simulink model "model"  (R2018a)
settings: Solver=FixedStepAuto  StartTime=0.0  StopTime=inf  FixedStep=0.1  MaxStep=0.1  MinStep=0.001  RelTol=1e-3
libraries: vrlib x19, simulink x15
(part 1 of 2)
settings Model: Creator=besho  LastModifiedBy=besho
settings SolverCC: ZeroCrossAlgorithm=Adaptive
settings DataIOCC: SaveOutput=off  SignalLogging=off  DSMLogging=off  SaveTime=off

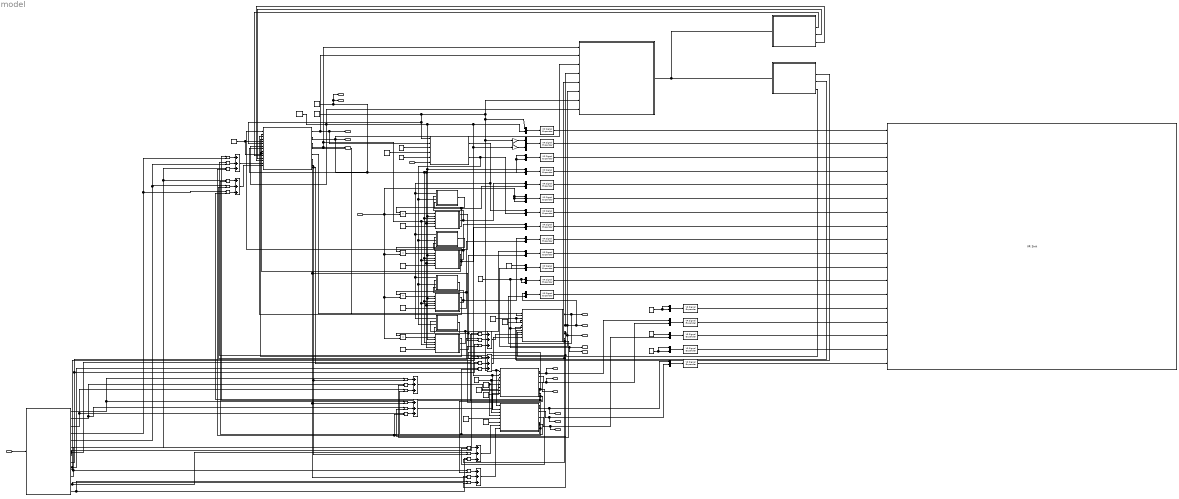
== system model ==
  light_switch : Inport
  light_moving : Inport  Port=2
  collision_matrix : Inport  Port=3  PortDimensions=[4 4]
  Add{,1..7} (8 alike) : Sum  Inputs=+++
  Bus Creator{,1..10,12..17} (17 alike) : BusCreator  Inputs=2
  Bus Creator11 : BusCreator  Inputs=3
  Constant{,1,6,11} (4 alike) : Constant  Value=0
  Constant10 : Constant  Value=200
  Constant{2,12,15..16} (4 alike) : Constant
  Constant13 : Constant  Value=4.7
  Constant14 : Constant  Value=100
  Constant3 : Constant  Value=3*pi/2
  Constant4 : Constant  Value=pi
  Constant5 : Constant  Value=pi/2
  Constant7 : Constant  Value=100
  Constant9 : Constant  Value=3
  Gain : Gain  Gain=1.1
  Gain1 : Gain  Gain=1.1
  MATLAB Function : MATLAB Function  TreatAsAtomicUnit=on
  Multiply{,1..27} (28 alike) : Product
  VR Signal Expander{,1..3,5..8,10,12..13,15..16} (13 alike) : vrlib/VR Signal Expander  outwidth=3  outidx=[1 2]
      settings: SourceProductName=Simulink 3D Animation  SourceProductBaseCode=VR
  VR Signal Expander11 : vrlib/VR Signal Expander  outwidth=3  outidx=[1 2 3]
      settings: SourceProductName=Simulink 3D Animation  SourceProductBaseCode=VR
  VR Signal Expander14 : vrlib/VR Signal Expander  outwidth=3  outidx=[1 3]
      settings: SourceProductName=Simulink 3D Animation  SourceProductBaseCode=VR
  VR Signal Expander17 : vrlib/VR Signal Expander  outwidth=4  outidx=[3 4]
      settings: SourceProductName=Simulink 3D Animation  SourceProductBaseCode=VR
  VR Signal Expander4 : vrlib/VR Signal Expander  outwidth=3  outidx=[1 3]
      settings: SourceProductName=Simulink 3D Animation  SourceProductBaseCode=VR
  VR Signal Expander9 : vrlib/VR Signal Expander  outwidth=4  outidx=[3 4]
      settings: SourceProductName=Simulink 3D Animation  SourceProductBaseCode=VR
  VR Sink : vrlib/VR Sink  InstantiateOnLoad=on  SampleTime=-1  ViewEnable=on  RemoteChange=off  RemoteView=off  FieldsWritten=arena.scale.3.1.1.double#out_of_bounds.scale.3.1.1.double#scout.scale.3.1.1.double#scout.translation.3.1.1.double#front_light_sensor.translation.3.1.1.double#light_spot.scale.3.1.1.double#light_spot.translation.3.1.1.double#back_light_sensor.translation.3.1.1.double#left_light_sensor.translation.3.1.1.double#right_light_sensor.translation.3.1.1.double#collector.rotation.4.1.1.double#collector.scale.3.1.1.double#collector.translation.3.1.1.double#opponent_scout.scale.3.1.1.double#opponent_scout.translation.3.1.1.double#opponent_collector.rotation.4.1.1.double#opponent_collector.scale.3.1.1.double#opponent_collector.translation.3.1.1.double  WorldFileName=visual.x3d  WorldDescription=Simulation  AutoView=off  VideoDimensions=[]  AllowVariableSize=off
      settings: SourceProductBaseCode=VR
  arena_x : Constant  Value=200
  arena_y : Constant  Value=100
  collector : Subsystem
  collector_receiver : Subsystem
  collector_side_length : Constant  Value=10
  collector_side_length1 : Constant  Value=10
  light_init_x : Constant  Value=100
  light_init_y : Constant  Value=50
  light_intensity_calculator_b : Subsystem
  light_intensity_calculator_f : Subsystem
  light_intensity_calculator_l : Subsystem
  light_intensity_calculator_r : Subsystem
  light_max_speed : Constant  Value=5
  light_spot : Subsystem
  ls_back : Subsystem
  ls_front : Subsystem
  ls_left : Subsystem
  ls_right : Subsystem
  opponent_collector : Subsystem
  opponent_scout : Subsystem
  referee : Subsystem
  scout : Subsystem
  scout_radius : Constant  Value=4.7
  scout_receiver : Subsystem
  scout_x : Outport
  scout_y : Outport  Port=2
  scout_theta : Outport  Port=3
  scout_r : Outport  Port=4
  collector_x : Outport  Port=5
  collector_y : Outport  Port=6
  collector_theta : Outport  Port=7
  collector_dimension : Outport  Port=8
  opp_scout_x : Outport  Port=9
  opp_scout_y : Outport  Port=10
  opp_scout_theta : Outport  Port=11
  opp_scout_r : Outport  Port=12
  opp_coll_x : Outport  Port=13
  opp_coll_y : Outport  Port=14
  opp_coll_theta : Outport  Port=15
  opp_collector_dimension : Outport  Port=16
  wires:
  Constant4/1 -> ls_back/6(offset)
  Constant1/1 -> ls_front/6(offset)
  Constant5/1 -> ls_left/6(offset)
  Constant3/1 -> ls_right/6(offset)
  scout/1(x) -> referee/2(scout_x), scout_x/1, Bus Creator/1, ls_back/2(scout_x_pos), ls_left/2(scout_x_pos), ls_right/2(scout_x_pos), ls_front/2(scout_x_pos)  "scout_x"
  scout/2(y) -> referee/3(scout_y), scout_y/1, ls_right/3(scout_y_pos), ls_left/3(scout_y_pos), ls_back/3(scout_y_pos), ls_front/3(scout_y_pos), Bus Creator/2  "scout_y"
  light_spot/1(x) -> Bus Creator1/1, light_intensity_calculator_r/1(light_spot_x), light_intensity_calculator_l/1(light_spot_x), light_intensity_calculator_b/1(light_spot_x), light_intensity_calculator_f/1(light_spot_x)  "light_x"
  Bus Creator1/1 -> VR Signal Expander5/1
  Gain/1 -> Bus Creator3/1
  Gain1/1 -> Bus Creator3/2
  Bus Creator3/1 -> VR Signal Expander/1
  Bus Creator5/1 -> VR Signal Expander1/1
  Bus Creator/1 -> VR Signal Expander3/1
  Bus Creator2/1 -> VR Signal Expander4/1
  Bus Creator4/1 -> VR Signal Expander2/1
  arena_x/1 -> opponent_collector/1(x_max), opponent_scout/1(x_max), Gain/1, Bus Creator4/1, referee/7(x_max), light_spot/1(x_max), scout/6(x_max)
  arena_y/1 -> opponent_collector/2(y_max), opponent_scout/2(y_max), Gain1/1, Bus Creator4/2, light_spot/2(y_max), referee/8(y_max), scout/7(y_max)
  light_max_speed/1 -> light_spot/3(speed_max)
  Bus Creator6/1 -> VR Signal Expander6/1
  Bus Creator7/1 -> VR Signal Expander7/1
  Bus Creator8/1 -> VR Signal Expander8/1
  ls_left/2(sensor_x_pos) -> light_intensity_calculator_l/2(light_sensor_x), Bus Creator7/1
  ls_left/3(sensor_y_pos) -> Bus Creator7/2, light_intensity_calculator_l/4(light_sensor_y)
  ls_right/2(sensor_x_pos) -> light_intensity_calculator_r/2(light_sensor_x), Bus Creator8/1
  ls_right/3(sensor_y_pos) -> light_intensity_calculator_r/4(light_sensor_y), Bus Creator8/2
  ls_front/2(sensor_x_pos) -> light_intensity_calculator_f/2(light_sensor_x), Bus Creator5/1
  ls_front/3(sensor_y_pos) -> Bus Creator5/2, light_intensity_calculator_f/4(light_sensor_y)
  ls_back/2(sensor_x_pos) -> Bus Creator6/1, light_intensity_calculator_b/2(light_sensor_x)
  ls_back/3(sensor_y_pos) -> Bus Creator6/2, light_intensity_calculator_b/4(light_sensor_y)
  scout_radius/1 -> opp_scout_r/1, scout_r/1, scout/8(scout_radius), ls_front/5(scout_radius), ls_right/5(scout_radius), ls_left/5(scout_radius), ls_back/5(scout_radius), Bus Creator2/1, Bus Creator2/2
  scout/3(orientation) -> ls_right/4(scout_orientation), ls_left/4(scout_orientation), ls_back/4(scout_orientation), ls_front/4(scout_orientation), referee/1(scout_theta), scout_theta/1
  light_spot/2(y) -> Bus Creator1/2, light_intensity_calculator_r/3(light_spot_y), light_intensity_calculator_l/3(light_spot_y), light_intensity_calculator_b/3(light_spot_y), light_intensity_calculator_f/3(light_spot_y)  "light_y"
  ls_front/1(sensor_out) -> scout/1(ls_f)
  ls_back/1(sensor_out) -> scout/2(ls_b)
  ls_left/1(sensor_out) -> scout/3(ls_l)
  ls_right/1(sensor_out) -> scout/4(ls_r)
  light_init_x/1 -> light_spot/4(x0)
  light_init_y/1 -> light_spot/5(y0)
  Constant/1 -> scout/10(x0), scout/9(y0), scout/5(theta0)
  light_intensity_calculator_f/1(light_intensity) -> Multiply/1
  light_switch/1 -> Multiply3/2, Multiply2/2, Multiply1/2, Bus Creator11/3, Bus Creator11/2, Bus Creator11/1, Multiply/2
  light_intensity_calculator_b/1(light_intensity) -> Multiply1/1
  light_intensity_calculator_l/1(light_intensity) -> Multiply2/1
  light_intensity_calculator_r/1(light_intensity) -> Multiply3/1
  Multiply3/1 -> ls_right/1(light_in)
  Multiply2/1 -> ls_left/1(light_in)
  Multiply1/1 -> ls_back/1(light_in)
  Multiply/1 -> ls_front/1(light_in)
  Bus Creator11/1 -> VR Signal Expander11/1
  light_moving/1 -> light_spot/6(move)
  Bus Creator9/1 -> VR Signal Expander9/1
  Constant2/1 -> Bus Creator9/1
  Bus Creator10/1 -> VR Signal Expander10/1
  Bus Creator12/1 -> VR Signal Expander12/1
  scout/4(x_dest) -> collector/1(x_scout)
  scout/5(y_dest) -> collector/2(y_scout)
  Constant6/1 -> collector/5(x0), collector/3(theta0)
  Constant7/1 -> collector/4(y0)
  collector_side_length/1 -> opp_collector_dimension/1, collector_dimension/1, collector/6(collector_side_length), Bus Creator12/2, Bus Creator12/1
  collector/2(x) -> collector_x/1, Bus Creator10/1, referee/4(collector_x)
  collector/1(y) -> collector_y/1, Bus Creator10/2, referee/5(collector_y)
  collector/3(theta) -> collector_theta/1, Bus Creator9/2, referee/6(collector_theta)
  referee/1(byte_out) -> scout_receiver/1(byte_in), collector_receiver/1(byte_in)
  scout_receiver/2(x) -> scout/11(referee_x)
  scout_receiver/3(y) -> scout/12(referee_y)
  scout_receiver/4(theta) -> scout/13(referee_theta)
  collector_receiver/3(y) -> collector/7(referee_y)
  collector_receiver/2(x) -> collector/8(referee_x)
  collector_receiver/4(theta) -> collector/9(referee_theta)
  Constant9/1 -> opponent_collector/3(speed_max), opponent_scout/3(speed_max)
  Constant10/1 -> opponent_collector/4(x0), opponent_scout/4(x0)
  Constant11/1 -> opponent_scout/5(y0)
  Constant12/1 -> opponent_scout/6(move)
  Bus Creator13/1 -> VR Signal Expander13/1
  opponent_scout/1(x) -> opp_scout_x/1, Bus Creator13/1
  opponent_scout/2(y) -> opp_scout_y/1, Bus Creator13/2
  Bus Creator14/1 -> VR Signal Expander14/1
  Constant13/1 -> Bus Creator14/1, Bus Creator14/2
  Constant14/1 -> opponent_collector/5(y0)
  Constant15/1 -> opponent_collector/6(move)
  Bus Creator15/1 -> VR Signal Expander15/1
  Bus Creator17/1 -> VR Signal Expander17/1
  Bus Creator16/1 -> VR Signal Expander16/1
  opponent_collector/1(x) -> opp_coll_x/1, Bus Creator15/1
  opponent_collector/2(y) -> opp_coll_y/1, Bus Creator15/2
  collector_side_length1/1 -> Bus Creator16/1, Bus Creator16/2
  Constant16/1 -> Bus Creator17/1
  opponent_collector/3(theta) -> opp_coll_theta/1, Bus Creator17/2
  VR Signal Expander2/1 -> VR Sink/1
  VR Signal Expander/1 -> VR Sink/2
  VR Signal Expander4/1 -> VR Sink/3
  VR Signal Expander3/1 -> VR Sink/4
  VR Signal Expander1/1 -> VR Sink/5
  VR Signal Expander11/1 -> VR Sink/6
  VR Signal Expander5/1 -> VR Sink/7
  VR Signal Expander6/1 -> VR Sink/8
  VR Signal Expander7/1 -> VR Sink/9
  VR Signal Expander8/1 -> VR Sink/10
  VR Signal Expander9/1 -> VR Sink/11
  VR Signal Expander12/1 -> VR Sink/12
  VR Signal Expander10/1 -> VR Sink/13
  VR Signal Expander17/1 -> VR Sink/16
  VR Signal Expander16/1 -> VR Sink/17
  VR Signal Expander15/1 -> VR Sink/18
  VR Signal Expander14/1 -> VR Sink/14
  VR Signal Expander13/1 -> VR Sink/15
  opponent_scout/3(theta) -> opp_scout_theta/1
  collision_matrix/1 -> MATLAB Function/1(u)
  Add/1 -> scout/14(dy_in)
  Add1/1 -> scout/15(dx_in)
  Multiply4/1 -> Add/1
  Multiply5/1 -> Add/2
  Multiply6/1 -> Add/3
  MATLAB Function/4(opsc_sc) -> Multiply9/1, Multiply4/2
  opponent_scout/5(dy) -> Multiply22/2, Multiply13/2, Multiply4/1
  MATLAB Function/5(col_sc) -> Multiply8/1, Multiply5/2
  collector/4(dy) -> Multiply20/2, Multiply5/1, Multiply15/2
  MATLAB Function/6(opcol_sc) -> Multiply7/1, Multiply6/1
  opponent_collector/5(dy) -> Multiply24/2, Multiply21/2, Multiply6/2
  Multiply7/1 -> Add1/1
  Multiply8/1 -> Add1/2
  Multiply9/1 -> Add1/3
  opponent_collector/4(dx) -> Multiply27/2, Multiply7/2, Multiply18/2
  collector/5(dx) -> Multiply17/2, Multiply12/2, Multiply8/2
  opponent_scout/4(dx) -> Multiply25/2, Multiply10/2, Multiply9/2
  Multiply11/1 -> Add2/2
  Multiply15/1 -> Add3/3
  Multiply14/1 -> Add3/2
  Multiply13/1 -> Add3/1
  Multiply12/1 -> Add2/3
  Multiply10/1 -> Add2/1
  Add2/1 -> opponent_collector/7(dx_in)
  scout/7(dx) -> Multiply26/2, Multiply16/2, Multiply11/2
  MATLAB Function/12(col_opcol) -> Multiply15/1, Multiply12/1
  Add3/1 -> opponent_collector/8(dy_in)
  scout/6(dy) -> Multiply23/2, Multiply19/2, Multiply14/2
  Multiply17/1 -> Add4/2
  Multiply21/1 -> Add5/3
  Multiply20/1 -> Add5/2
  Multiply19/1 -> Add5/1
  Multiply18/1 -> Add4/3
  Multiply16/1 -> Add4/1
  Add4/1 -> opponent_scout/7(dx_in)
  MATLAB Function/1(sc_opsc) -> Multiply19/1, Multiply16/1
  MATLAB Function/2(col_opsc) -> Multiply20/1, Multiply17/1
  MATLAB Function/3(opcol_opsc) -> Multiply21/1, Multiply18/1
  Add5/1 -> opponent_scout/8(dy_in)
  Multiply23/1 -> Add6/2
  Multiply27/1 -> Add7/3
  Multiply26/1 -> Add7/2
  Multiply25/1 -> Add7/1
  Multiply24/1 -> Add6/3
  Multiply22/1 -> Add6/1
  Add6/1 -> collector/10(dy_in)
  MATLAB Function/9(opcol_col) -> Multiply27/1, Multiply24/1
  Add7/1 -> collector/11(dx_in)
  MATLAB Function/7(opsc_col) -> Multiply25/1, Multiply22/1
  MATLAB Function/8(sc_col) -> Multiply26/1, Multiply23/1
  MATLAB Function/10(opsc_opcol) -> Multiply13/1, Multiply10/1
  MATLAB Function/11(sc_opcol) -> Multiply14/1, Multiply11/1

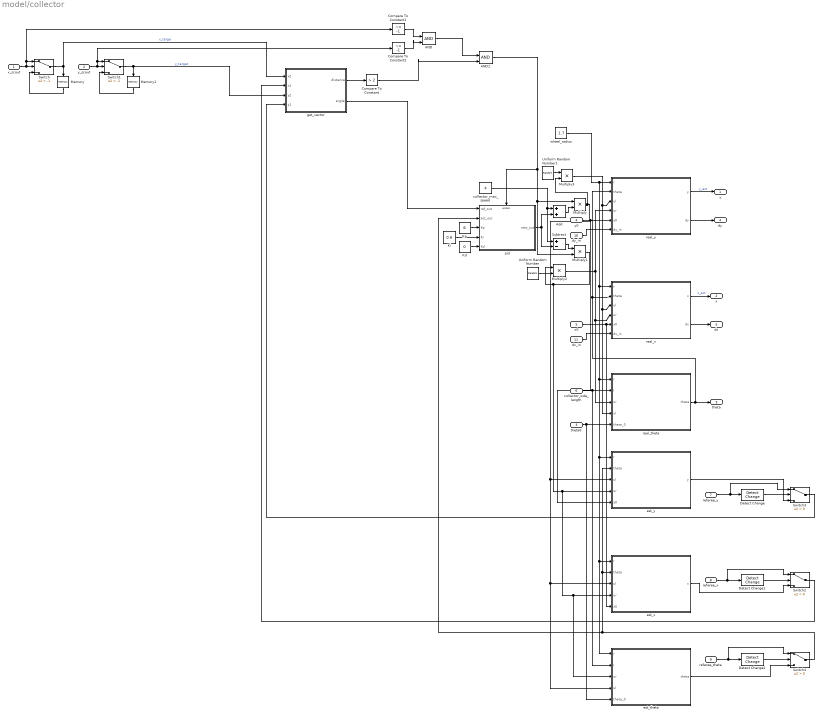
== system model/collector ==
  x_scout : Inport
  y_scout : Inport  Port=2
  theta0 : Inport  Port=3
  y0 : Inport  Port=4
  x0 : Inport  Port=5
  collector_side_length : Inport  Port=6
  referee_y : Inport  Port=7
  referee_x : Inport  Port=8
  referee_theta : Inport  Port=9
  dy_in : Inport  Port=10
  dx_in : Inport  Port=11
  AND : Logic  IconShape=distinctive  AllPortsSameDT=off  OutDataTypeStr=boolean
  AND1 : Logic  IconShape=distinctive  AllPortsSameDT=off  OutDataTypeStr=boolean
  Add : Sum
  Compare To Constant : simulink/Logic and Bit Operations/Compare To Constant  relop=>  const=2  OutDataTypeStr=boolean
  Compare To Constant1 : simulink/Logic and Bit Operations/Compare To Constant  relop=~=  const=-1  OutDataTypeStr=boolean
  Compare To Constant2 : simulink/Logic and Bit Operations/Compare To Constant  relop=~=  const=-1  OutDataTypeStr=boolean
  Detect Change : simulink/Logic and Bit Operations/Detect Change  vinit=100  OutDataTypeStr=boolean
  Detect Change1 : simulink/Logic and Bit Operations/Detect Change  vinit=0  OutDataTypeStr=boolean
  Detect Change2 : simulink/Logic and Bit Operations/Detect Change  vinit=0  OutDataTypeStr=boolean
  Kd : Constant  Value=0
  Ki : Constant  Value=0.6
  Kp : Constant  Value=6
  Memory : Memory
  Memory1 : Memory
  Multiply{,1..3} (4 alike) : Product
  Subtract : Sum  Inputs=+-
  Switch : Switch  Criteria=u2 > Threshold  Threshold=-1
  Switch1 : Switch  Criteria=u2 > Threshold  Threshold=-1
  Switch2 : Switch  Criteria=u2 > Threshold
  Switch3 : Switch  Criteria=u2 > Threshold
  Switch4 : Switch  Criteria=u2 > Threshold
  Uniform Random Number : UniformRandomNumber  Minimum=0.98  Maximum=1.02  Seed=170  SampleTime=0.1
  Uniform Random Number1 : UniformRandomNumber  Minimum=0.98  Maximum=1.02  Seed=4  SampleTime=0.1
  collector_max_speed : Constant  Value=4
  est_theta : Subsystem
  est_x : Subsystem
  est_y : Subsystem
  get_vector : Subsystem
  pid : Subsystem
  real_theta : Subsystem
  real_x : Subsystem
  real_y : Subsystem
  wheel_radius : Constant  Value=1.7
  y : Outport
  x : Outport  Port=2
  theta : Outport  Port=3
  dy : Outport  Port=4
  dx : Outport  Port=5
  wires:
  wheel_radius/1 -> est_theta/1(r), est_x/1(r), est_y/1(r), real_theta/1(r), real_x/1(r), real_y/1(r)
  Memory1/1 -> Switch1/3
  x0/1 -> est_x/5(x0), real_x/5(x0)
  Compare To Constant2/1 -> AND/2
  AND/1 -> AND1/1
  Switch/1 -> get_vector/1(x2), Memory/1  "x_targe"
  get_vector/2(angle) -> pid/1(ref_out)
  y_scout/1 -> Compare To Constant2/1, Switch1/1, Switch1/2
  Memory/1 -> Switch/3
  y0/1 -> est_y/5(y0), real_y/5(y0)
  x_scout/1 -> Compare To Constant1/1, Switch/1, Switch/2
  Kp/1 -> pid/3(Kp)
  Switch1/1 -> Memory1/1, get_vector/3(y2)  "y_target"
  real_theta/1(theta) -> theta/1, real_y/2(theta), real_x/2(theta)
  Ki/1 -> pid/4(Ki)
  Kd/1 -> pid/5(Kd)
  collector_max_speed/1 -> Subtract/1, Add/1
  Compare To Constant1/1 -> AND/1
  real_y/1(y) -> y/1  "y_act"
  pid/1(new_out) -> Add/2, Subtract/2
  Compare To Constant/1 -> AND1/2
  AND1/1 -> pid/Enable, Multiply1/2, Multiply/1
  get_vector/1(distance) -> Compare To Constant/1
  theta0/1 -> est_theta/5(theta_0), real_theta/5(theta_0)
  real_x/1(x) -> x/1  "x_act"
  Uniform Random Number/1 -> Multiply2/2
  Uniform Random Number1/1 -> Multiply3/1
  collector_side_length/1 -> real_theta/2(l), est_theta/2(l)
  Switch4/1 -> pid/2(act_out), est_y/2(theta), est_x/2(theta)
  Switch3/1 -> get_vector/4(y1)
  Switch2/1 -> get_vector/2(x1)
  Add/1 -> Multiply/2
  Multiply/1 -> est_theta/4(ul), est_x/3(ul), est_y/3(ul), Multiply3/2
  Subtract/1 -> Multiply1/1
  Multiply1/1 -> est_theta/3(ur), est_x/4(ur), est_y/4(ur), Multiply2/1
  Multiply2/1 -> real_y/4(ur), real_theta/3(ur), real_x/4(ur)
  Multiply3/1 -> real_y/3(ul), real_x/3(ul), real_theta/4(ul)
  referee_y/1 -> Switch3/1, Detect Change/1
  Detect Change/1 -> Switch3/2
  est_y/1(y) -> Switch3/3
  referee_x/1 -> Switch2/1, Detect Change1/1
  Detect Change1/1 -> Switch2/2
  est_x/1(x) -> Switch2/3
  referee_theta/1 -> Switch4/1, Detect Change2/1
  Detect Change2/1 -> Switch4/2
  est_theta/1(theta) -> Switch4/3
  real_y/2(dy) -> dy/1
  real_x/2(dx) -> dx/1
  dy_in/1 -> real_y/6(dy_in)
  dx_in/1 -> real_x/6(dx_in)

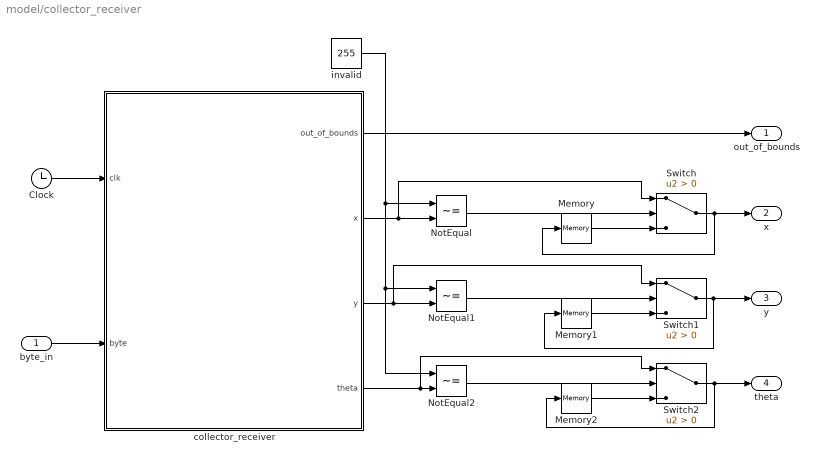
== system model/collector_receiver ==
  byte_in : Inport
  Clock : Clock
  Memory : Memory
  Memory1 : Memory
  Memory2 : Memory
  NotEqual : RelationalOperator  Operator=~=  OutDataTypeStr=boolean  RndMeth=Simplest
  NotEqual1 : RelationalOperator  Operator=~=  OutDataTypeStr=boolean  RndMeth=Simplest
  NotEqual2 : RelationalOperator  Operator=~=  OutDataTypeStr=boolean  RndMeth=Simplest
  Switch : Switch  Criteria=u2 > Threshold
  Switch1 : Switch  Criteria=u2 > Threshold
  Switch2 : Switch  Criteria=u2 > Threshold
  collector_receiver : MATLAB Function  TreatAsAtomicUnit=on
  invalid : Constant  Value=255
  out_of_bounds : Outport
  x : Outport  Port=2
  y : Outport  Port=3
  theta : Outport  Port=4
  wires:
  byte_in/1 -> collector_receiver/2(byte)
  Memory2/1 -> Switch2/3
  collector_receiver/4(theta) -> NotEqual2/2, Switch2/1
  Switch1/1 -> Memory1/1, y/1
  Memory1/1 -> Switch1/3
  Memory/1 -> Switch/3
  NotEqual/1 -> Switch/2
  collector_receiver/2(x) -> NotEqual/2, Switch/1
  invalid/1 -> NotEqual2/1, NotEqual1/1, NotEqual/1
  collector_receiver/1(out_of_bounds) -> out_of_bounds/1
  Switch2/1 -> Memory2/1, theta/1
  NotEqual2/1 -> Switch2/2
  Switch/1 -> Memory/1, x/1
  Clock/1 -> collector_receiver/1(clk)
  NotEqual1/1 -> Switch1/2
  collector_receiver/3(y) -> NotEqual1/2, Switch1/1

== system model/light_intensity_calculator_b ==
  light_spot_x : Inport
  light_sensor_x : Inport  Port=2
  light_spot_y : Inport  Port=3
  light_sensor_y : Inport  Port=4
  Max : MinMax  Function=max  Inputs=2
  Minus : Sum  Inputs=-+
  Multiply : Product
  Terminator : Terminator
  get_vector : Subsystem
  light_min_intensity : Constant  Value=0
  light_spot_degradation_factor : Constant  Value=20
  light_spot_max_intensity : Constant  Value=255
  light_intensity : Outport
  wires:
  get_vector/2(angle) -> Terminator/1
  Max/1 -> light_intensity/1
  light_min_intensity/1 -> Max/2
  light_sensor_x/1 -> get_vector/2(x1)
  Minus/1 -> Max/1
  Multiply/1 -> Minus/1
  light_spot_y/1 -> get_vector/3(y2)
  light_spot_degradation_factor/1 -> Multiply/1
  light_spot_max_intensity/1 -> Minus/2
  get_vector/1(distance) -> Multiply/2
  light_sensor_y/1 -> get_vector/4(y1)
  light_spot_x/1 -> get_vector/1(x2)

== system model/light_intensity_calculator_f ==
  light_spot_x : Inport
  light_sensor_x : Inport  Port=2
  light_spot_y : Inport  Port=3
  light_sensor_y : Inport  Port=4
  Max : MinMax  Function=max  Inputs=2
  Minus : Sum  Inputs=-+
  Multiply : Product
  Terminator : Terminator
  get_vector : Subsystem
  light_min_intensity : Constant  Value=0
  light_spot_degradation_factor : Constant  Value=20
  light_spot_max_intensity : Constant  Value=255
  light_intensity : Outport
  wires:
  light_spot_x/1 -> get_vector/1(x2)
  light_sensor_y/1 -> get_vector/4(y1)
  get_vector/1(distance) -> Multiply/2
  light_spot_max_intensity/1 -> Minus/2
  light_spot_degradation_factor/1 -> Multiply/1
  light_spot_y/1 -> get_vector/3(y2)
  Multiply/1 -> Minus/1
  Minus/1 -> Max/1
  light_sensor_x/1 -> get_vector/2(x1)
  light_min_intensity/1 -> Max/2
  Max/1 -> light_intensity/1
  get_vector/2(angle) -> Terminator/1

== system model/light_intensity_calculator_l ==
  light_spot_x : Inport
  light_sensor_x : Inport  Port=2
  light_spot_y : Inport  Port=3
  light_sensor_y : Inport  Port=4
  Max : MinMax  Function=max  Inputs=2
  Minus : Sum  Inputs=-+
  Multiply : Product
  Terminator : Terminator
  get_vector : Subsystem
  light_min_intensity : Constant  Value=0
  light_spot_degradation_factor : Constant  Value=20
  light_spot_max_intensity : Constant  Value=255
  light_intensity : Outport
  wires:
  light_spot_x/1 -> get_vector/1(x2)
  light_sensor_y/1 -> get_vector/4(y1)
  get_vector/1(distance) -> Multiply/2
  light_spot_max_intensity/1 -> Minus/2
  light_spot_degradation_factor/1 -> Multiply/1
  light_spot_y/1 -> get_vector/3(y2)
  Multiply/1 -> Minus/1
  Minus/1 -> Max/1
  light_sensor_x/1 -> get_vector/2(x1)
  light_min_intensity/1 -> Max/2
  Max/1 -> light_intensity/1
  get_vector/2(angle) -> Terminator/1

== system model/light_intensity_calculator_r ==
  light_spot_x : Inport
  light_sensor_x : Inport  Port=2
  light_spot_y : Inport  Port=3
  light_sensor_y : Inport  Port=4
  Max : MinMax  Function=max  Inputs=2
  Minus : Sum  Inputs=-+
  Multiply : Product
  Terminator : Terminator
  get_vector : Subsystem
  light_min_intensity : Constant  Value=0
  light_spot_degradation_factor : Constant  Value=20
  light_spot_max_intensity : Constant  Value=255
  light_intensity : Outport
  wires:
  get_vector/2(angle) -> Terminator/1
  Max/1 -> light_intensity/1
  light_min_intensity/1 -> Max/2
  light_sensor_x/1 -> get_vector/2(x1)
  Minus/1 -> Max/1
  Multiply/1 -> Minus/1
  light_spot_y/1 -> get_vector/3(y2)
  light_spot_degradation_factor/1 -> Multiply/1
  light_spot_max_intensity/1 -> Minus/2
  get_vector/1(distance) -> Multiply/2
  light_sensor_y/1 -> get_vector/4(y1)
  light_spot_x/1 -> get_vector/1(x2)

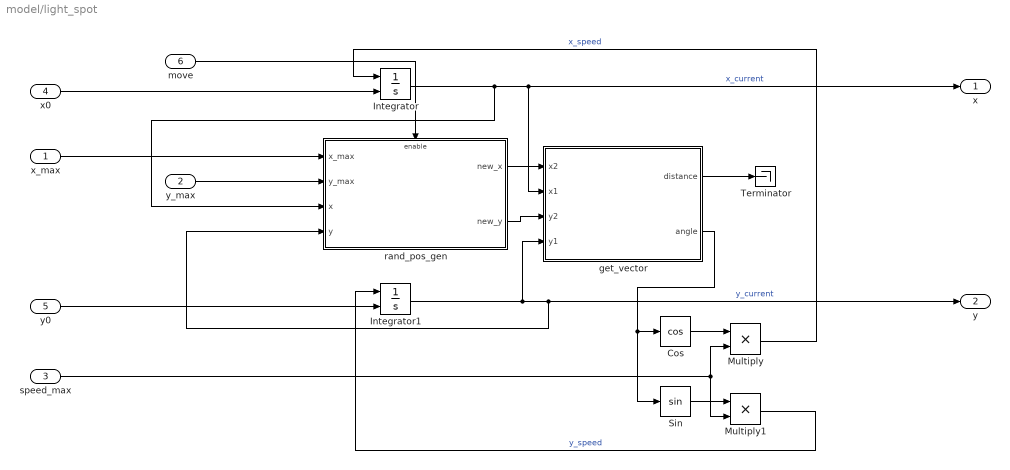
== system model/light_spot ==
  x_max : Inport
  y_max : Inport  Port=2
  speed_max : Inport  Port=3
  x0 : Inport  Port=4
  y0 : Inport  Port=5
  move : Inport  Port=6
  Cos : Trigonometry  Operator=cos
  Integrator : Integrator  InitialConditionSource=external
  Integrator1 : Integrator  InitialConditionSource=external
  Multiply : Product
  Multiply1 : Product
  Sin : Trigonometry
  Terminator : Terminator
  get_vector : Subsystem
  rand_pos_gen : Subsystem
  x : Outport
  y : Outport  Port=2
  wires:
  Multiply1/1 -> Integrator1/1  "y_speed"
  Multiply/1 -> Integrator/1  "x_speed"
  Integrator/1 -> rand_pos_gen/3(x), x/1, get_vector/2(x1)  "x_current"
  x0/1 -> Integrator/2
  Sin/1 -> Multiply1/1
  Cos/1 -> Multiply/1
  Integrator1/1 -> get_vector/4(y1), y/1, rand_pos_gen/4(y)  "y_current"
  speed_max/1 -> Multiply/2, Multiply1/2
  y0/1 -> Integrator1/2
  x_max/1 -> rand_pos_gen/1(x_max)
  y_max/1 -> rand_pos_gen/2(y_max)
  rand_pos_gen/1(new_x) -> get_vector/1(x2)
  rand_pos_gen/2(new_y) -> get_vector/3(y2)
  get_vector/1(distance) -> Terminator/1
  get_vector/2(angle) -> Sin/1, Cos/1
  move/1 -> rand_pos_gen/Enable

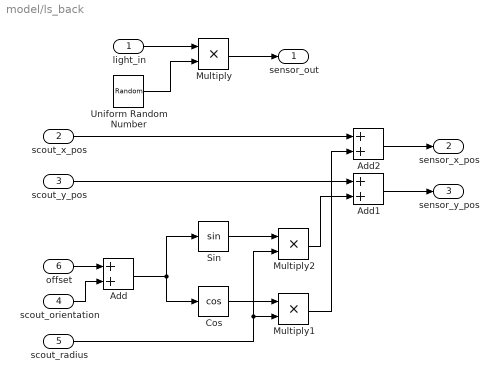
== system model/ls_back ==
  light_in : Inport
  scout_x_pos : Inport  Port=2
  scout_y_pos : Inport  Port=3
  scout_orientation : Inport  Port=4
  scout_radius : Inport  Port=5
  offset : Inport  Port=6
  Add : Sum
  Add1 : Sum
  Add2 : Sum
  Cos : Trigonometry  Operator=cos
  Multiply : Product
  Multiply1 : Product
  Multiply2 : Product
  Sin : Trigonometry
  Uniform Random Number : UniformRandomNumber  Minimum=0.96  Maximum=1.04  Seed=68  SampleTime=0.1
  sensor_out : Outport
  sensor_x_pos : Outport  Port=2
  sensor_y_pos : Outport  Port=3
  wires:
  Uniform Random Number/1 -> Multiply/2
  Multiply/1 -> sensor_out/1
  light_in/1 -> Multiply/1
  scout_orientation/1 -> Add/2
  Cos/1 -> Multiply1/1
  scout_radius/1 -> Multiply2/2, Multiply1/2
  Sin/1 -> Multiply2/1
  offset/1 -> Add/1
  Add/1 -> Cos/1, Sin/1
  scout_x_pos/1 -> Add2/1
  Multiply1/1 -> Add2/2
  scout_y_pos/1 -> Add1/1
  Multiply2/1 -> Add1/2
  Add2/1 -> sensor_x_pos/1
  Add1/1 -> sensor_y_pos/1

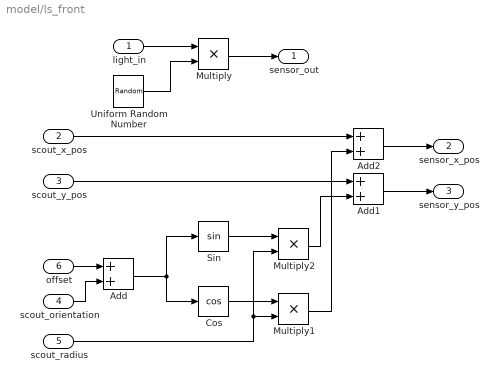
== system model/ls_front ==
  light_in : Inport
  scout_x_pos : Inport  Port=2
  scout_y_pos : Inport  Port=3
  scout_orientation : Inport  Port=4
  scout_radius : Inport  Port=5
  offset : Inport  Port=6
  Add : Sum
  Add1 : Sum
  Add2 : Sum
  Cos : Trigonometry  Operator=cos
  Multiply : Product
  Multiply1 : Product
  Multiply2 : Product
  Sin : Trigonometry
  Uniform Random Number : UniformRandomNumber  Minimum=0.96  Maximum=1.04  Seed=24  SampleTime=0.1
  sensor_out : Outport
  sensor_x_pos : Outport  Port=2
  sensor_y_pos : Outport  Port=3
  wires:
  Uniform Random Number/1 -> Multiply/2
  Multiply/1 -> sensor_out/1
  light_in/1 -> Multiply/1
  scout_orientation/1 -> Add/2
  Cos/1 -> Multiply1/1
  scout_radius/1 -> Multiply2/2, Multiply1/2
  Sin/1 -> Multiply2/1
  offset/1 -> Add/1
  Add/1 -> Cos/1, Sin/1
  scout_x_pos/1 -> Add2/1
  Multiply1/1 -> Add2/2
  scout_y_pos/1 -> Add1/1
  Multiply2/1 -> Add1/2
  Add2/1 -> sensor_x_pos/1
  Add1/1 -> sensor_y_pos/1

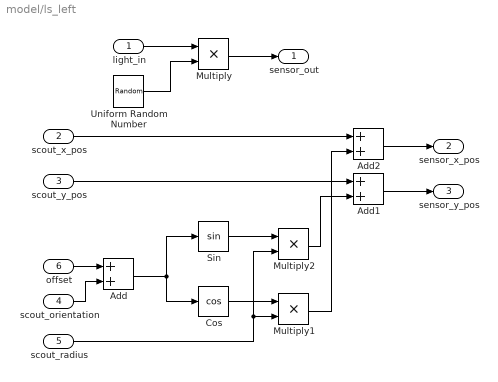
== system model/ls_left ==
  light_in : Inport
  scout_x_pos : Inport  Port=2
  scout_y_pos : Inport  Port=3
  scout_orientation : Inport  Port=4
  scout_radius : Inport  Port=5
  offset : Inport  Port=6
  Add : Sum
  Add1 : Sum
  Add2 : Sum
  Cos : Trigonometry  Operator=cos
  Multiply : Product
  Multiply1 : Product
  Multiply2 : Product
  Sin : Trigonometry
  Uniform Random Number : UniformRandomNumber  Minimum=0.96  Maximum=1.04  Seed=105  SampleTime=0.1
  sensor_out : Outport
  sensor_x_pos : Outport  Port=2
  sensor_y_pos : Outport  Port=3
  wires:
  Uniform Random Number/1 -> Multiply/2
  Multiply/1 -> sensor_out/1
  light_in/1 -> Multiply/1
  scout_orientation/1 -> Add/2
  Cos/1 -> Multiply1/1
  scout_radius/1 -> Multiply2/2, Multiply1/2
  Sin/1 -> Multiply2/1
  offset/1 -> Add/1
  Add/1 -> Cos/1, Sin/1
  scout_x_pos/1 -> Add2/1
  Multiply1/1 -> Add2/2
  scout_y_pos/1 -> Add1/1
  Multiply2/1 -> Add1/2
  Add2/1 -> sensor_x_pos/1
  Add1/1 -> sensor_y_pos/1

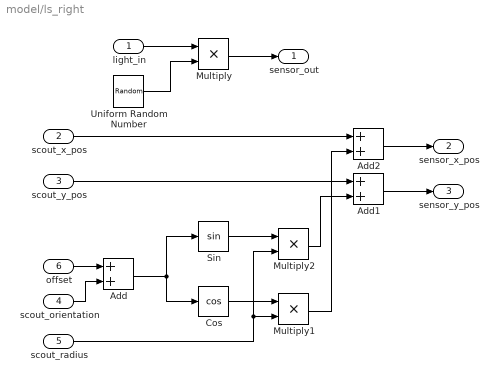
== system model/ls_right ==
  light_in : Inport
  scout_x_pos : Inport  Port=2
  scout_y_pos : Inport  Port=3
  scout_orientation : Inport  Port=4
  scout_radius : Inport  Port=5
  offset : Inport  Port=6
  Add : Sum
  Add1 : Sum
  Add2 : Sum
  Cos : Trigonometry  Operator=cos
  Multiply : Product
  Multiply1 : Product
  Multiply2 : Product
  Sin : Trigonometry
  Uniform Random Number : UniformRandomNumber  Minimum=0.96  Maximum=1.04  Seed=189  SampleTime=0.1
  sensor_out : Outport
  sensor_x_pos : Outport  Port=2
  sensor_y_pos : Outport  Port=3
  wires:
  Uniform Random Number/1 -> Multiply/2
  Multiply/1 -> sensor_out/1
  light_in/1 -> Multiply/1
  scout_orientation/1 -> Add/2
  Cos/1 -> Multiply1/1
  scout_radius/1 -> Multiply2/2, Multiply1/2
  Sin/1 -> Multiply2/1
  offset/1 -> Add/1
  Add/1 -> Cos/1, Sin/1
  scout_x_pos/1 -> Add2/1
  Multiply1/1 -> Add2/2
  scout_y_pos/1 -> Add1/1
  Multiply2/1 -> Add1/2
  Add2/1 -> sensor_x_pos/1
  Add1/1 -> sensor_y_pos/1

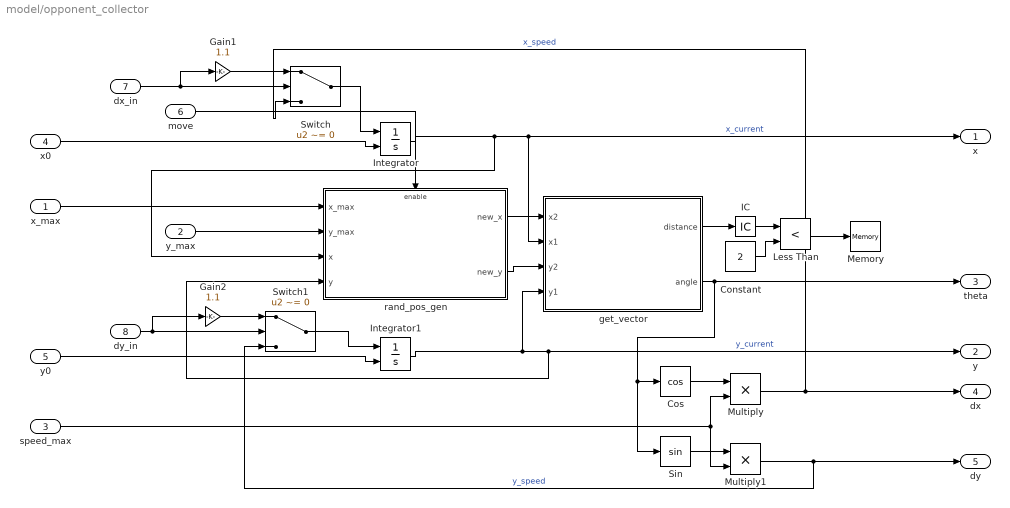
== system model/opponent_collector ==
  x_max : Inport
  y_max : Inport  Port=2
  speed_max : Inport  Port=3
  x0 : Inport  Port=4
  y0 : Inport  Port=5
  move : Inport  Port=6
  dx_in : Inport  Port=7
  dy_in : Inport  Port=8
  Constant : Constant  Value=2
  Cos : Trigonometry  Operator=cos
  Gain1 : Gain  Gain=1.1
  Gain2 : Gain  Gain=1.1
  IC : InitialCondition  Value=0
  Integrator : Integrator  InitialConditionSource=external
  Integrator1 : Integrator  InitialConditionSource=external
  Less Than : RelationalOperator  Operator=<  OutDataTypeStr=boolean  RndMeth=Simplest
  Memory : Memory
  Multiply : Product
  Multiply1 : Product
  Sin : Trigonometry
  Switch : Switch  Criteria=u2 ~= 0
  Switch1 : Switch  Criteria=u2 ~= 0
  get_vector : Subsystem
  rand_pos_gen : Subsystem
  x : Outport
  y : Outport  Port=2
  theta : Outport  Port=3
  dx : Outport  Port=4
  dy : Outport  Port=5
  wires:
  Multiply1/1 -> Switch1/3, dy/1  "y_speed"
  Multiply/1 -> Switch/3, dx/1  "x_speed"
  Integrator/1 -> rand_pos_gen/3(x), x/1, get_vector/2(x1)  "x_current"
  x0/1 -> Integrator/2
  Sin/1 -> Multiply1/1
  Cos/1 -> Multiply/1
  Integrator1/1 -> get_vector/4(y1), y/1, rand_pos_gen/4(y)  "y_current"
  speed_max/1 -> Multiply/2, Multiply1/2
  y0/1 -> Integrator1/2
  x_max/1 -> rand_pos_gen/1(x_max)
  y_max/1 -> rand_pos_gen/2(y_max)
  rand_pos_gen/1(new_x) -> get_vector/1(x2)
  rand_pos_gen/2(new_y) -> get_vector/3(y2)
  get_vector/2(angle) -> theta/1, Sin/1, Cos/1
  move/1 -> rand_pos_gen/Enable
  dx_in/1 -> Switch/2, Gain1/1
  Switch/1 -> Integrator/1
  dy_in/1 -> Switch1/2, Gain2/1
  Switch1/1 -> Integrator1/1
  Gain1/1 -> Switch/1
  Gain2/1 -> Switch1/1
  get_vector/1(distance) -> IC/1
  IC/1 -> Less Than/1
  Constant/1 -> Less Than/2
  Less Than/1 -> Memory/1

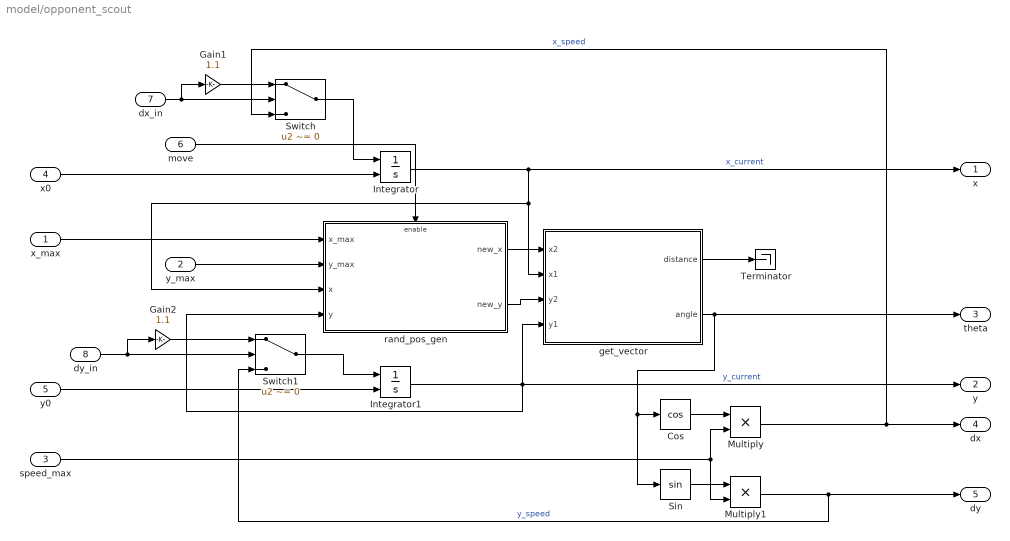
== system model/opponent_scout ==
  x_max : Inport
  y_max : Inport  Port=2
  speed_max : Inport  Port=3
  x0 : Inport  Port=4
  y0 : Inport  Port=5
  move : Inport  Port=6
  dx_in : Inport  Port=7
  dy_in : Inport  Port=8
  Cos : Trigonometry  Operator=cos
  Gain1 : Gain  Gain=1.1
  Gain2 : Gain  Gain=1.1
  Integrator : Integrator  InitialConditionSource=external
  Integrator1 : Integrator  InitialConditionSource=external
  Multiply : Product
  Multiply1 : Product
  Sin : Trigonometry
  Switch : Switch  Criteria=u2 ~= 0
  Switch1 : Switch  Criteria=u2 ~= 0
  Terminator : Terminator
  get_vector : Subsystem
  rand_pos_gen : Subsystem
  x : Outport
  y : Outport  Port=2
  theta : Outport  Port=3
  dx : Outport  Port=4
  dy : Outport  Port=5
  wires:
  Multiply1/1 -> Switch1/3, dy/1  "y_speed"
  Multiply/1 -> Switch/3, dx/1  "x_speed"
  Integrator/1 -> rand_pos_gen/3(x), get_vector/2(x1), x/1  "x_current"
  x0/1 -> Integrator/2
  Sin/1 -> Multiply1/1
  Cos/1 -> Multiply/1
  Integrator1/1 -> y/1, rand_pos_gen/4(y), get_vector/4(y1)  "y_current"
  speed_max/1 -> Multiply/2, Multiply1/2
  y0/1 -> Integrator1/2
  x_max/1 -> rand_pos_gen/1(x_max)
  y_max/1 -> rand_pos_gen/2(y_max)
  rand_pos_gen/1(new_x) -> get_vector/1(x2)
  rand_pos_gen/2(new_y) -> get_vector/3(y2)
  get_vector/1(distance) -> Terminator/1
  get_vector/2(angle) -> theta/1, Sin/1, Cos/1
  move/1 -> rand_pos_gen/Enable
  dx_in/1 -> Switch/2, Gain1/1
  Switch/1 -> Integrator/1
  dy_in/1 -> Switch1/2, Gain2/1
  Switch1/1 -> Integrator1/1
  Gain1/1 -> Switch/1
  Gain2/1 -> Switch1/1

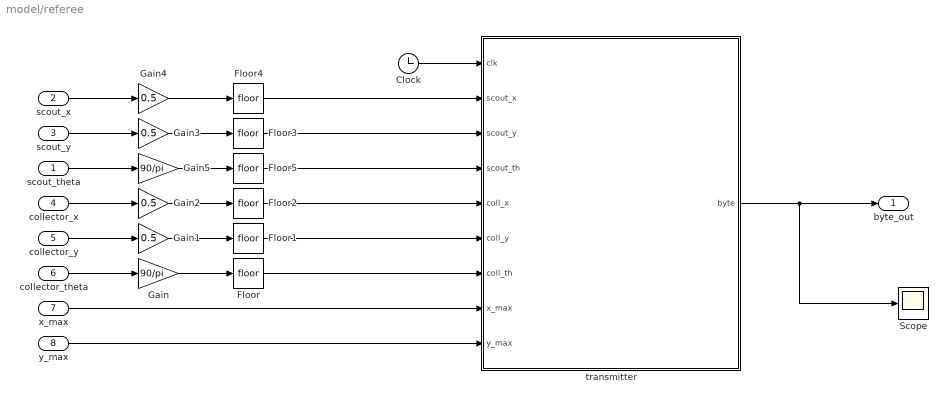
== system model/referee ==
  scout_theta : Inport
  scout_x : Inport  Port=2
  scout_y : Inport  Port=3
  collector_x : Inport  Port=4
  collector_y : Inport  Port=5
  collector_theta : Inport  Port=6
  x_max : Inport  Port=7
  y_max : Inport  Port=8
  Clock : Clock
  Floor{,1..5} (6 alike) : Rounding
  Gain : Gain  Gain=90/pi
  Gain{1..4} (4 alike) : Gain  Gain=0.5
  Gain5 : Gain  Gain=90/pi
  Scope : Scope
  transmitter : MATLAB Function  TreatAsAtomicUnit=on
  byte_out : Outport
  wires:
  transmitter/1(byte) -> Scope/1, byte_out/1
  Floor2/1 -> transmitter/5(coll_x)
  Floor1/1 -> transmitter/6(coll_y)
  y_max/1 -> transmitter/9(y_max)
  scout_theta/1 -> Gain5/1
  Gain5/1 -> Floor5/1
  x_max/1 -> transmitter/8(x_max)
  Floor3/1 -> transmitter/3(scout_y)
  Floor/1 -> transmitter/7(coll_th)
  Gain/1 -> Floor/1
  Clock/1 -> transmitter/1(clk)
  Floor5/1 -> transmitter/4(scout_th)
  Floor4/1 -> transmitter/2(scout_x)
  collector_x/1 -> Gain2/1
  Gain4/1 -> Floor4/1
  collector_y/1 -> Gain1/1
  collector_theta/1 -> Gain/1
  Gain2/1 -> Floor2/1
  scout_x/1 -> Gain4/1
  Gain1/1 -> Floor1/1
  Gain3/1 -> Floor3/1
  scout_y/1 -> Gain3/1

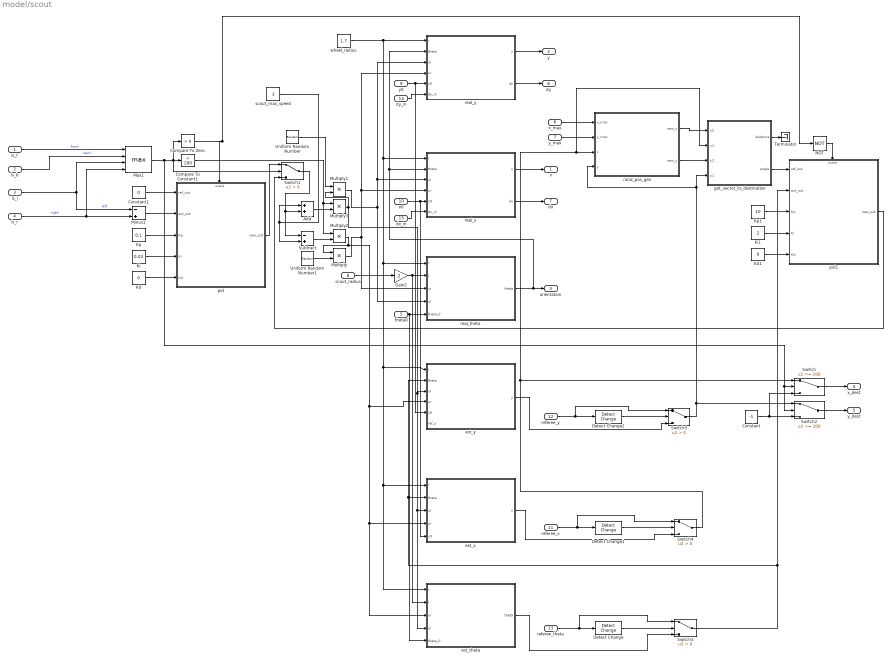
== system model/scout ==
  ls_f : Inport
  ls_b : Inport  Port=2
  ls_l : Inport  Port=3
  ls_r : Inport  Port=4
  theta0 : Inport  Port=5
  x_max : Inport  Port=6
  y_max : Inport  Port=7
  scout_radius : Inport  Port=8
  y0 : Inport  Port=9
  x0 : Inport  Port=10
  referee_x : Inport  Port=11
  referee_y : Inport  Port=12
  referee_theta : Inport  Port=13
  dy_in : Inport  Port=14
  dx_in : Inport  Port=15
  Add : Sum
  Compare To Constant1 : simulink/Logic and Bit Operations/Compare To Constant  relop=<  const=200  OutDataTypeStr=boolean
  Compare To Zero : simulink/Logic and Bit Operations/Compare To Zero  relop=>  OutDataTypeStr=boolean
  Constant : Constant  Value=-1
  Constant1 : Constant  Value=0
  Detect Change : simulink/Logic and Bit Operations/Detect Change  vinit=0  OutDataTypeStr=boolean
  Detect Change1 : simulink/Logic and Bit Operations/Detect Change  vinit=0  OutDataTypeStr=boolean
  Detect Change2 : simulink/Logic and Bit Operations/Detect Change  vinit=0  OutDataTypeStr=boolean
  Gain2 : Gain  Gain=2
  Kd : Constant  Value=0
  Kd1 : Constant  Value=0
  Ki : Constant  Value=0.02
  Ki1 : Constant  Value=2
  Kp : Constant  Value=0.1
  Kp1 : Constant  Value=10
  Max1 : MinMax  Function=max  Inputs=4
  Minus1 : Sum  Inputs=-+
  Multiply{,1..3} (4 alike) : Product
  NOT : Logic  Operator=NOT  IconShape=distinctive  AllPortsSameDT=off  OutDataTypeStr=boolean
  Subtract : Sum  Inputs=-+
  Switch : Switch  Threshold=200
  Switch{1,3..5} (4 alike) : Switch  Criteria=u2 > Threshold
  Switch2 : Switch  Threshold=200
  Terminator : Terminator
  Uniform Random Number : UniformRandomNumber  Minimum=0.98  Maximum=1.02  Seed=69  SampleTime=0.1
  Uniform Random Number1 : UniformRandomNumber  Minimum=0.98  Maximum=1.02  Seed=25  SampleTime=0.1
  est_theta : Subsystem
  est_x : Subsystem
  est_y : Subsystem
  get_vector_to_destination : Subsystem
  pid : Subsystem
  pid1 : Subsystem
  rand_pos_gen : Subsystem
  real_theta : Subsystem
  real_x : Subsystem
  real_y : Subsystem
  scout_max_speed : Constant  Value=3
  wheel_radius : Constant  Value=1.7
  x : Outport
  y : Outport  Port=2
  orientation : Outport  Port=3
  x_dest : Outport  Port=4
  y_dest : Outport  Port=5
  dy : Outport  Port=6
  dx : Outport  Port=7
  wires:
  Add/1 -> Multiply3/2
  Subtract/1 -> Multiply2/2
  Multiply1/1 -> real_theta/4(ul), real_y/3(ul), real_x/3(ul)
  Multiply/1 -> real_theta/3(ur), real_y/4(ur), real_x/4(ur)
  wheel_radius/1 -> est_theta/1(r), est_x/1(r), est_y/1(r), real_theta/1(r), real_x/1(r), real_y/1(r)
  y0/1 -> est_y/5(y0), real_y/5(y0)
  x0/1 -> est_x/5(x0), real_x/5(x0)
  theta0/1 -> real_theta/5(theta_0), est_theta/5(theta_0)
  Gain2/1 -> est_theta/2(l), real_theta/2(l)
  scout_radius/1 -> Gain2/1
  real_y/1(y) -> y/1
  real_x/1(x) -> x/1
  ls_f/1 -> Max1/1  "front"
  ls_b/1 -> Max1/2  "back"
  ls_l/1 -> Max1/3, Minus1/1  "left"
  ls_r/1 -> Max1/4, Minus1/2  "right"
  Kp/1 -> pid/3(Kp)
  Kd/1 -> pid/5(Kd)
  Ki/1 -> pid/4(Ki)
  real_theta/1(theta) -> real_y/2(theta), real_x/2(theta), orientation/1
  Constant1/1 -> pid/1(ref_out)
  Minus1/1 -> pid/2(act_out)
  scout_max_speed/1 -> Add/1, Subtract/2
  x_max/1 -> rand_pos_gen/1(x_max)
  y_max/1 -> rand_pos_gen/2(y_max)
  rand_pos_gen/1(new_x) -> get_vector_to_destination/1(x2)
  rand_pos_gen/2(new_y) -> get_vector_to_destination/3(y2)
  get_vector_to_destination/2(angle) -> pid1/1(ref_out)
  Kd1/1 -> pid1/5(Kd)
  Ki1/1 -> pid1/4(Ki)
  Kp1/1 -> pid1/3(Kp)
  Compare To Constant1/1 -> Multiply2/1, Multiply3/1
  Max1/1 -> Switch2/2, Switch/2, Compare To Zero/1, Switch1/2, Compare To Constant1/1
  pid/1(new_out) -> Switch1/1
  Switch1/1 -> Add/2, Subtract/1
  pid1/1(new_out) -> Switch1/3
  NOT/1 -> pid1/Enable
  Compare To Zero/1 -> pid/Enable, NOT/1
  get_vector_to_destination/1(distance) -> Terminator/1
  Multiply2/1 -> est_theta/3(ur), est_x/4(ur), est_y/4(ur), Multiply/1
  Uniform Random Number1/1 -> Multiply/2
  Multiply3/1 -> est_theta/4(ul), est_x/3(ul), est_y/3(ul), Multiply1/2
  Uniform Random Number/1 -> Multiply1/1
  Switch3/1 -> est_y/2(theta), est_x/2(theta), pid1/2(act_out)
  Switch4/1 -> Switch/1, rand_pos_gen/3(x), get_vector_to_destination/2(x1)
  Switch5/1 -> Switch2/1, rand_pos_gen/4(y), get_vector_to_destination/4(y1)
  Switch/1 -> x_dest/1
  Switch2/1 -> y_dest/1
  Constant/1 -> Switch/3, Switch2/3
  referee_theta/1 -> Switch3/1, Detect Change/1
  Detect Change/1 -> Switch3/2
  est_theta/1(theta) -> Switch3/3
  referee_x/1 -> Switch4/1, Detect Change1/1
  Detect Change1/1 -> Switch4/2
  est_x/1(x) -> Switch4/3
  referee_y/1 -> Switch5/1, Detect Change2/1
  Detect Change2/1 -> Switch5/2
  est_y/1(y) -> Switch5/3
  real_y/2(dy) -> dy/1
  real_x/2(dx) -> dx/1
  dy_in/1 -> real_y/6(dy_in)
  dx_in/1 -> real_x/6(dx_in)

== system model/scout_receiver ==
  byte_in : Inport
  Clock : Clock
  Memory : Memory
  Memory1 : Memory
  Memory2 : Memory
  NotEqual : RelationalOperator  Operator=~=  OutDataTypeStr=boolean  RndMeth=Simplest
  NotEqual1 : RelationalOperator  Operator=~=  OutDataTypeStr=boolean  RndMeth=Simplest
  NotEqual2 : RelationalOperator  Operator=~=  OutDataTypeStr=boolean  RndMeth=Simplest
  Switch : Switch  Criteria=u2 > Threshold
  Switch1 : Switch  Criteria=u2 > Threshold
  Switch2 : Switch  Criteria=u2 > Threshold
  invalid : Constant  Value=255
  scout_receiver : MATLAB Function  TreatAsAtomicUnit=on
  out_of_bounds : Outport
  x : Outport  Port=2
  y : Outport  Port=3
  theta : Outport  Port=4
  wires:
  scout_receiver/3(y) -> Switch1/1, NotEqual1/2
  NotEqual1/1 -> Switch1/2
  Clock/1 -> scout_receiver/1(clk)
  Switch/1 -> x/1, Memory/1
  NotEqual2/1 -> Switch2/2
  Switch2/1 -> theta/1, Memory2/1
  scout_receiver/1(out_of_bounds) -> out_of_bounds/1
  invalid/1 -> NotEqual/1, NotEqual1/1, NotEqual2/1
  scout_receiver/2(x) -> Switch/1, NotEqual/2
  NotEqual/1 -> Switch/2
  Memory/1 -> Switch/3
  Memory1/1 -> Switch1/3
  Switch1/1 -> y/1, Memory1/1
  scout_receiver/4(theta) -> Switch2/1, NotEqual2/2
  Memory2/1 -> Switch2/3
  byte_in/1 -> scout_receiver/2(byte)

== system model/collector/est_theta ==
  r : Inport
  l : Inport  Port=2
  ur : Inport  Port=3
  ul : Inport  Port=4
  theta_0 : Inport  Port=5
  Divide : Product  Inputs=**/
  Integrator : Integrator  InitialConditionSource=external
  Minus : Sum  Inputs=+-
  theta : Outport
  wires:
  theta_0/1 -> Integrator/2
  ur/1 -> Minus/2
  l/1 -> Divide/3
  Minus/1 -> Divide/2
  r/1 -> Divide/1
  ul/1 -> Minus/1
  Integrator/1 -> theta/1
  Divide/1 -> Integrator/1

== system model/collector/est_x ==
  r : Inport
  theta : Inport  Port=2
  ul : Inport  Port=3
  ur : Inport  Port=4
  x0 : Inport  Port=5
  Add : Sum
  Cos : Trigonometry  Operator=cos
  Gain : Gain  Gain=1/2
  Integrator : Integrator  InitialConditionSource=external
  Multiply : Product  Inputs=3
  x : Outport
  wires:
  r/1 -> Multiply/1
  ur/1 -> Add/2
  Add/1 -> Multiply/2
  theta/1 -> Cos/1
  Cos/1 -> Multiply/3
  Integrator/1 -> x/1
  Multiply/1 -> Gain/1
  ul/1 -> Add/1
  Gain/1 -> Integrator/1
  x0/1 -> Integrator/2

== system model/collector/est_y ==
  r : Inport
  theta : Inport  Port=2
  ul : Inport  Port=3
  ur : Inport  Port=4
  y0 : Inport  Port=5
  Add : Sum
  Cos : Trigonometry
  Gain : Gain  Gain=1/2
  Integrator : Integrator  InitialConditionSource=external
  Multiply : Product  Inputs=3
  y : Outport
  wires:
  r/1 -> Multiply/1
  ur/1 -> Add/2
  Add/1 -> Multiply/2
  theta/1 -> Cos/1
  Cos/1 -> Multiply/3
  Integrator/1 -> y/1
  Multiply/1 -> Gain/1
  ul/1 -> Add/1
  Gain/1 -> Integrator/1
  y0/1 -> Integrator/2

== system model/collector/get_vector ==
  x2 : Inport
  x1 : Inport  Port=2
  y2 : Inport  Port=3
  y1 : Inport  Port=4
  Add : Sum
  Atan2 : Trigonometry  Operator=atan2
  Minus : Sum  Inputs=+-
  Minus1 : Sum  Inputs=+-
  Sqrt : Sqrt  SaturateOnIntegerOverflow=on
  Square : Math  Operator=square  SaturateOnIntegerOverflow=on
  Square1 : Math  Operator=square  SaturateOnIntegerOverflow=on
  distance : Outport
  angle : Outport  Port=2
  wires:
  Minus/1 -> Atan2/2, Square1/1
  y1/1 -> Minus1/2
  Square/1 -> Add/2
  Minus1/1 -> Atan2/1, Square/1
  Add/1 -> Sqrt/1
  Square1/1 -> Add/1
  x1/1 -> Minus/2
  x2/1 -> Minus/1
  Sqrt/1 -> distance/1
  y2/1 -> Minus1/1
  Atan2/1 -> angle/1

== system model/collector/pid ==
  ref_out : Inport
  act_out : Inport  Port=2
  Kp : Inport  Port=3
  Ki : Inport  Port=4
  Kd : Inport  Port=5
  Enable : EnablePort  StatesWhenEnabling=reset
  Discrete Derivative : simulink/Discrete/Discrete Derivative  gainval=1.0  ICPrevScaledInput=0.0  OutMin=[]  OutMax=[]  OutDataType=fixdt(1, 16)  OutScaling=2^-10  DoSatur=off
  Integrator : Integrator
  Multiply : Product
  Multiply1 : Product
  Multiply2 : Product
  Sum : Sum  Inputs=|+-
  Sum1 : Sum  Inputs=+++
  new_out : Outport
  wires:
  act_out/1 -> Sum/2
  Ki/1 -> Multiply1/2
  Multiply/1 -> Sum1/1
  Kd/1 -> Multiply2/2
  Sum/1 -> Multiply/1, Integrator/1, Discrete Derivative/1
  Kp/1 -> Multiply/2
  ref_out/1 -> Sum/1
  Integrator/1 -> Multiply1/1
  Multiply1/1 -> Sum1/2
  Multiply2/1 -> Sum1/3
  Sum1/1 -> new_out/1
  Discrete Derivative/1 -> Multiply2/1

== system model/collector/real_theta ==
  r : Inport
  l : Inport  Port=2
  ur : Inport  Port=3
  ul : Inport  Port=4
  theta_0 : Inport  Port=5
  Divide : Product  Inputs=**/
  Integrator : Integrator  InitialConditionSource=external
  Minus : Sum  Inputs=+-
  theta : Outport
  wires:
  theta_0/1 -> Integrator/2
  ur/1 -> Minus/2
  l/1 -> Divide/3
  Minus/1 -> Divide/2
  r/1 -> Divide/1
  ul/1 -> Minus/1
  Integrator/1 -> theta/1
  Divide/1 -> Integrator/1

== system model/collector/real_x ==
  r : Inport
  theta : Inport  Port=2
  ul : Inport  Port=3
  ur : Inport  Port=4
  x0 : Inport  Port=5
  dx_in : Inport  Port=6
  Add : Sum
  Cos : Trigonometry  Operator=cos
  Gain : Gain  Gain=1/2
  Gain1 : Gain  Gain=1.1
  Integrator : Integrator  InitialConditionSource=external
  Multiply : Product  Inputs=3
  Switch : Switch  Criteria=u2 ~= 0
  x : Outport
  dx : Outport  Port=2
  wires:
  r/1 -> Multiply/1
  ur/1 -> Add/2
  Add/1 -> Multiply/2
  theta/1 -> Cos/1
  Cos/1 -> Multiply/3
  Integrator/1 -> x/1
  Multiply/1 -> Gain/1
  ul/1 -> Add/1
  Gain/1 -> Switch/3, dx/1
  x0/1 -> Integrator/2
  dx_in/1 -> Switch/2, Gain1/1
  Switch/1 -> Integrator/1
  Gain1/1 -> Switch/1

== system model/collector/real_y ==
  r : Inport
  theta : Inport  Port=2
  ul : Inport  Port=3
  ur : Inport  Port=4
  y0 : Inport  Port=5
  dy_in : Inport  Port=6
  Add : Sum
  Cos : Trigonometry
  Gain : Gain  Gain=1/2
  Gain1 : Gain  Gain=1.1
  Integrator : Integrator  InitialConditionSource=external
  Multiply : Product  Inputs=3
  Switch : Switch  Criteria=u2 ~= 0
  y : Outport
  dy : Outport  Port=2
  wires:
  r/1 -> Multiply/1
  ur/1 -> Add/2
  Add/1 -> Multiply/2
  theta/1 -> Cos/1
  Cos/1 -> Multiply/3
  Integrator/1 -> y/1
  Multiply/1 -> Gain/1
  ul/1 -> Add/1
  Gain/1 -> Switch/3, dy/1
  y0/1 -> Integrator/2
  dy_in/1 -> Switch/2, Gain1/1
  Switch/1 -> Integrator/1
  Gain1/1 -> Switch/1

== system model/light_intensity_calculator_b/get_vector ==
  x2 : Inport
  x1 : Inport  Port=2
  y2 : Inport  Port=3
  y1 : Inport  Port=4
  Add : Sum
  Atan2 : Trigonometry  Operator=atan2
  Minus : Sum  Inputs=+-
  Minus1 : Sum  Inputs=+-
  Sqrt : Sqrt  SaturateOnIntegerOverflow=on
  Square : Math  Operator=square  SaturateOnIntegerOverflow=on
  Square1 : Math  Operator=square  SaturateOnIntegerOverflow=on
  distance : Outport
  angle : Outport  Port=2
  wires:
  Atan2/1 -> angle/1
  y2/1 -> Minus1/1
  Sqrt/1 -> distance/1
  x2/1 -> Minus/1
  x1/1 -> Minus/2
  Square1/1 -> Add/1
  Add/1 -> Sqrt/1
  Minus1/1 -> Square/1, Atan2/1
  Square/1 -> Add/2
  y1/1 -> Minus1/2
  Minus/1 -> Square1/1, Atan2/2

== system model/light_intensity_calculator_f/get_vector ==
  x2 : Inport
  x1 : Inport  Port=2
  y2 : Inport  Port=3
  y1 : Inport  Port=4
  Add : Sum
  Atan2 : Trigonometry  Operator=atan2
  Minus : Sum  Inputs=+-
  Minus1 : Sum  Inputs=+-
  Sqrt : Sqrt  SaturateOnIntegerOverflow=on
  Square : Math  Operator=square  SaturateOnIntegerOverflow=on
  Square1 : Math  Operator=square  SaturateOnIntegerOverflow=on
  distance : Outport
  angle : Outport  Port=2
  wires:
  Minus/1 -> Atan2/2, Square1/1
  y1/1 -> Minus1/2
  Square/1 -> Add/2
  Minus1/1 -> Atan2/1, Square/1
  Add/1 -> Sqrt/1
  Square1/1 -> Add/1
  x1/1 -> Minus/2
  x2/1 -> Minus/1
  Sqrt/1 -> distance/1
  y2/1 -> Minus1/1
  Atan2/1 -> angle/1

== system model/light_intensity_calculator_l/get_vector ==
  x2 : Inport
  x1 : Inport  Port=2
  y2 : Inport  Port=3
  y1 : Inport  Port=4
  Add : Sum
  Atan2 : Trigonometry  Operator=atan2
  Minus : Sum  Inputs=+-
  Minus1 : Sum  Inputs=+-
  Sqrt : Sqrt  SaturateOnIntegerOverflow=on
  Square : Math  Operator=square  SaturateOnIntegerOverflow=on
  Square1 : Math  Operator=square  SaturateOnIntegerOverflow=on
  distance : Outport
  angle : Outport  Port=2
  wires:
  Minus/1 -> Atan2/2, Square1/1
  y1/1 -> Minus1/2
  Square/1 -> Add/2
  Minus1/1 -> Atan2/1, Square/1
  Add/1 -> Sqrt/1
  Square1/1 -> Add/1
  x1/1 -> Minus/2
  x2/1 -> Minus/1
  Sqrt/1 -> distance/1
  y2/1 -> Minus1/1
  Atan2/1 -> angle/1

== system model/light_intensity_calculator_r/get_vector ==
  x2 : Inport
  x1 : Inport  Port=2
  y2 : Inport  Port=3
  y1 : Inport  Port=4
  Add : Sum
  Atan2 : Trigonometry  Operator=atan2
  Minus : Sum  Inputs=+-
  Minus1 : Sum  Inputs=+-
  Sqrt : Sqrt  SaturateOnIntegerOverflow=on
  Square : Math  Operator=square  SaturateOnIntegerOverflow=on
  Square1 : Math  Operator=square  SaturateOnIntegerOverflow=on
  distance : Outport
  angle : Outport  Port=2
  wires:
  Atan2/1 -> angle/1
  y2/1 -> Minus1/1
  Sqrt/1 -> distance/1
  x2/1 -> Minus/1
  x1/1 -> Minus/2
  Square1/1 -> Add/1
  Add/1 -> Sqrt/1
  Minus1/1 -> Square/1, Atan2/1
  Square/1 -> Add/2
  y1/1 -> Minus1/2
  Minus/1 -> Square1/1, Atan2/2

== system model/light_spot/get_vector ==
  x2 : Inport
  x1 : Inport  Port=2
  y2 : Inport  Port=3
  y1 : Inport  Port=4
  Add : Sum
  Atan2 : Trigonometry  Operator=atan2
  Minus : Sum  Inputs=+-
  Minus1 : Sum  Inputs=+-
  Sqrt : Sqrt  SaturateOnIntegerOverflow=on
  Square : Math  Operator=square  SaturateOnIntegerOverflow=on
  Square1 : Math  Operator=square  SaturateOnIntegerOverflow=on
  distance : Outport
  angle : Outport  Port=2
  wires:
  Minus/1 -> Atan2/2, Square1/1
  y1/1 -> Minus1/2
  Square/1 -> Add/2
  Minus1/1 -> Atan2/1, Square/1
  Add/1 -> Sqrt/1
  Square1/1 -> Add/1
  x1/1 -> Minus/2
  x2/1 -> Minus/1
  Sqrt/1 -> distance/1
  y2/1 -> Minus1/1
  Atan2/1 -> angle/1

== system model/light_spot/rand_pos_gen ==
  x_max : Inport
  y_max : Inport  Port=2
  x : Inport  Port=3
  y : Inport  Port=4
  Enable : EnablePort
  Constant : Constant  Value=2
  IC : InitialCondition  Value=0
  Less Than : RelationalOperator  Operator=<  OutDataTypeStr=boolean  RndMeth=Simplest
  Memory : Memory
  Terminator : Terminator
  get_vector : Subsystem
  rand_position_gen : Subsystem
  new_x : Outport
  new_y : Outport  Port=2
  wires:
  get_vector/2(angle) -> Terminator/1
  y/1 -> get_vector/4(y1)
  Less Than/1 -> Memory/1
  Memory/1 -> rand_position_gen/Trigger
  x_max/1 -> rand_position_gen/1(x_max)
  x/1 -> get_vector/2(x1)
  rand_position_gen/1(x_out) -> new_x/1, get_vector/1(x2)
  rand_position_gen/2(y_out) -> new_y/1, get_vector/3(y2)
  y_max/1 -> rand_position_gen/2(y_max)
  Constant/1 -> Less Than/2
  get_vector/1(distance) -> IC/1
  IC/1 -> Less Than/1

== system model/opponent_collector/get_vector ==
  x2 : Inport
  x1 : Inport  Port=2
  y2 : Inport  Port=3
  y1 : Inport  Port=4
  Add : Sum
  Atan2 : Trigonometry  Operator=atan2
  Minus : Sum  Inputs=+-
  Minus1 : Sum  Inputs=+-
  Sqrt : Sqrt  SaturateOnIntegerOverflow=on
  Square : Math  Operator=square  SaturateOnIntegerOverflow=on
  Square1 : Math  Operator=square  SaturateOnIntegerOverflow=on
  distance : Outport
  angle : Outport  Port=2
  wires:
  Minus/1 -> Atan2/2, Square1/1
  y1/1 -> Minus1/2
  Square/1 -> Add/2
  Minus1/1 -> Atan2/1, Square/1
  Add/1 -> Sqrt/1
  Square1/1 -> Add/1
  x1/1 -> Minus/2
  x2/1 -> Minus/1
  Sqrt/1 -> distance/1
  y2/1 -> Minus1/1
  Atan2/1 -> angle/1

== system model/opponent_collector/rand_pos_gen ==
  x_max : Inport
  y_max : Inport  Port=2
  x : Inport  Port=3
  y : Inport  Port=4
  Enable : EnablePort
  Constant : Constant  Value=2
  IC : InitialCondition  Value=0
  Less Than : RelationalOperator  Operator=<  OutDataTypeStr=boolean  RndMeth=Simplest
  Memory : Memory
  Terminator : Terminator
  get_vector : Subsystem
  rand_position_gen : Subsystem
  new_x : Outport
  new_y : Outport  Port=2
  wires:
  get_vector/2(angle) -> Terminator/1
  y/1 -> get_vector/4(y1)
  Less Than/1 -> Memory/1
  Memory/1 -> rand_position_gen/Trigger
  x_max/1 -> rand_position_gen/1(x_max)
  x/1 -> get_vector/2(x1)
  rand_position_gen/1(x_out) -> new_x/1, get_vector/1(x2)
  get_vector/1(distance) -> IC/1
  rand_position_gen/2(y_out) -> new_y/1, get_vector/3(y2)
  y_max/1 -> rand_position_gen/2(y_max)
  Constant/1 -> Less Than/2
  IC/1 -> Less Than/1

== system model/opponent_scout/get_vector ==
  x2 : Inport
  x1 : Inport  Port=2
  y2 : Inport  Port=3
  y1 : Inport  Port=4
  Add : Sum
  Atan2 : Trigonometry  Operator=atan2
  Minus : Sum  Inputs=+-
  Minus1 : Sum  Inputs=+-
  Sqrt : Sqrt  SaturateOnIntegerOverflow=on
  Square : Math  Operator=square  SaturateOnIntegerOverflow=on
  Square1 : Math  Operator=square  SaturateOnIntegerOverflow=on
  distance : Outport
  angle : Outport  Port=2
  wires:
  Minus/1 -> Atan2/2, Square1/1
  y1/1 -> Minus1/2
  Square/1 -> Add/2
  Minus1/1 -> Atan2/1, Square/1
  Add/1 -> Sqrt/1
  Square1/1 -> Add/1
  x1/1 -> Minus/2
  x2/1 -> Minus/1
  Sqrt/1 -> distance/1
  y2/1 -> Minus1/1
  Atan2/1 -> angle/1
